simulink model "sdruFMMono"  (Simulink 8.1)
settings: Solver=FixedStepDiscrete  SolverMode=SingleTasking  StartTime=0.0  StopTime=inf  RelTol=1e-3
PreLoadFcn:
  | monoFM = getParamsSdruFMMonoDemo;
InitFcn:
  | monoFM = getParamsSdruFMMonoDemo;
undefined symbols (not defined in the file or in its folder): mfilt
libraries: simulink x1, dspmlti4 x1, dsparch4 x1, dspsigops x1, dspsnks4 x1, sdrublksprivate x1, commsdrhw_v2 x1
Description:
  | This model uses Universal Software Radio Peripheral (USRP) hardware with Simulink(R) to perform FM mono demodulation.
CloseFcn:
  | clear monoFM
settings Model: Creator=The MathWorks Inc.
settings DataIOCC: SaveOutput=off  SignalLogging=off  DSMLogging=off  SaveTime=off
settings OptimizationCC: SimCompilerOptimization=On
settings DebuggingCC: InheritedTsInSrcMsg=none  MultiTaskCondExecSysMsg=none  ParameterPrecisionLossMsg=none
settings HardwareCC: TargetBitPerLong=64  TargetBitPerPointer=64  TargetIntDivRoundTo=Zero  TargetEndianess=LittleEndian  TargetWordSize=64  TargetHWDeviceType=Generic->MATLAB Host Computer  ProdEqTarget=off
settings SFSimCC: SFSimEnableDebug=off  SFSimOverflowDetection=off  SimIntegrity=off
settings RTWCC: CustomSourceCode=|
  | #include <stdio.h>
  | #include <stdlib.h>

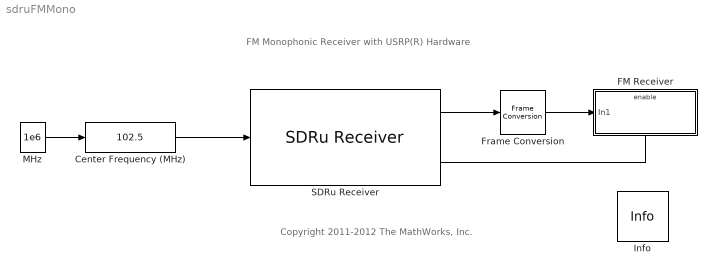
== system sdruFMMono ==
  note: FM Monophonic Receiver with USRP(R) Hardware
  note: Copyright 2011-2012 The MathWorks, Inc.
  Center Frequency (MHz) : simulink/Math Operations/Slider Gain  low=87.5  gain=102.5  high=108
  FM Receiver : Subsystem  TreatAsAtomicUnit=on
  Frame Conversion : FrameConversion
  Info : sdrublksprivate/Info  SystemSampleTime=-1
  MHz : Constant  Value=1e6  VectorParams1D=off  SampleTime=-1  FramePeriod=-1
  SDRu Receiver : commsdrhw_v2/SDRu Receiver  rxtx=rx  USRP2_IP='192.168.10.2'  centerFrequency=2.45e9  centerFrequencySrc=Input port  loOffset=0  loOffsetSrc=Dialog  gain=monoFM.USRPGaindB  gainSrc=Dialog  decimInterp=monoFM.USRPDecimationFactor  decimInterpSrc=Dialog  USRP2_IP_NUM=[49 57 50 46 49 54 56 46 49 48 46 50]  frameLength=monoFM.FrameLength  outputDatatype=single  overrunUnderrunPort=off  sampleTime=1/monoFM.Fs  HOST_DATA_PORT=30000  HOST_CONTROL_PORT=30002  USRP2_DATA_PORT=32769  USRP2_CONTROL_PORT=32768  bufferMode=Continuous streaming  EnableBurstMode=off  NumFramesInBurst=100
  wires:
  Center Frequency (MHz)/1 -> SDRu Receiver/1
  SDRu Receiver/2 -> FM Receiver/Enable
  MHz/1 -> Center Frequency (MHz)/1
  SDRu Receiver/1 -> Frame Conversion/1
  Frame Conversion/1 -> FM Receiver/1(In1)

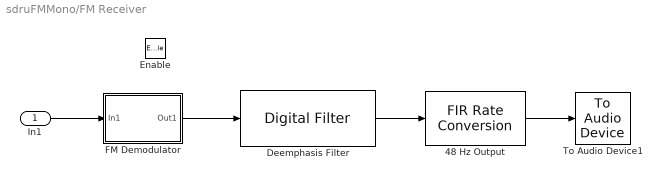
== system sdruFMMono/FM Receiver ==
  In1 : Inport
  Enable : EnablePort
  48 Hz Output : dspmlti4/FIR Rate Conversion  L=monoFM.InterpolationFactor  h=monoFM.Lowpass15k  M=monoFM.DecimationFactor  firstCoeffDataTypeStr=Inherit: Same word length as input  firstCoeffLastDataTypeStr=Inherit: Same word length as input  firstCoeffMin=[]  firstCoeffMax=[]  outputDataTypeStr=Inherit: Same as accumulator  outputLastDataTypeStr=Inherit: Same as accumulator  outputMin=[]  outputMax=[]  roundingMode=Floor  overflowMode=off  FilterSource=Specify via dialog  FilterObject=mfilt.firsrc(6,5)
  Deemphasis Filter : dsparch4/Digital Filter  TypePopup=IIR (poles & zeros)  IIRFiltStruct=Direct form II transposed  AllPoleFiltStruct=Direct form  FIRFiltStruct=Direct form  CoeffSource=Specify via dialog  NumCoeffs=[1 2]  DenCoeffs=[1 0.1]  BiQuadCoeffs=[1 0.3 0.4 1 0.1 0.2]  LatticeCoeffs=[0.2 0.4]  denIgnore=on  FiltPerSampPopup=One filter per frame  IC=0  ICnum=0  ICden=0  roundingMode=Floor  overflowMode=off  ScaleValues=1  scaleValueFracLength=14  stageInFracLength=15  stageOutFracLength=15  FilterSource=dfilt object  dfiltObjectName=monoFM.DeemphasisFilter  InputProcessing=Columns as channels (frame based)
  FM Demodulator : Subsystem
  To Audio Device1 : dspsnks4/To Audio Device  deviceName=Default  inheritSampleRate=on  sampleRate=48009  deviceDatatype=Determine from input data type  autoBufferSize=on  bufferSize=4096  queueDuration=1.0
  wires:
  FM Demodulator/1(Out1) -> Deemphasis Filter/1
  Deemphasis Filter/1 -> 48 Hz Output/1
  In1/1 -> FM Demodulator/1(In1)
  48 Hz Output/1 -> To Audio Device1/1

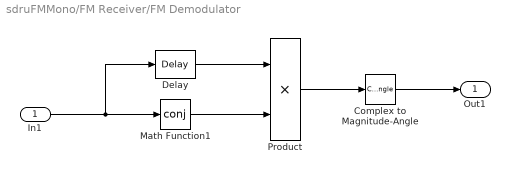
== system sdruFMMono/FM Receiver/FM Demodulator ==
  In1 : Inport
  Complex to Magnitude-Angle : ComplexToMagnitudeAngle  Output=Angle
  Delay : dspsigops/Delay  InputProcessing=Columns as channels (frame based)  dly_unit=Samples  delay=1  ic_detail=off  dif_ic_for_ch=off  dif_ic_for_dly=off  ic=0  reset_popup=None
  Math Function1 : Math  Operator=conj  SaturateOnIntegerOverflow=on
  Product : Product  RndMeth=Zero
  Out1 : Outport
  wires:
  Product/1 -> Complex to Magnitude-Angle/1
  Delay/1 -> Product/1
  In1/1 -> Delay/1, Math Function1/1
  Math Function1/1 -> Product/2
  Complex to Magnitude-Angle/1 -> Out1/1
